simulink model "Q8"  (R2017a)
settings: Solver=ode4  StartTime=0.0  StopTime=10000  FixedStep=0.01  RelTol=1e-3  EnableMultiTasking=on
undefined symbols (not defined in the file): Cg, Cs, k, kc, kg, kr, sCon, Ta, u0
settings Model: Creator=Mikkel  LastModifiedBy=pebark
settings DataIOCC: LimitDataPoints=on  SaveFormat=Array  SignalLoggingSaveFormat=ModelDataLogs
settings OptimizationCC: ExpressionDepthLimit=2147483647  LifeSpan=inf
settings DebuggingCC: UnderspecifiedInitializationDetection=Classic  MergeDetectMultiDrivingBlocksExec=none  SolverPrmCheckMsg=warning  FcnCallInpInsideContextMsg=warning  StateNameClashWarn=warning  SFUnexpectedBacktrackingDiag=warning  SFNoUnconditionalDefaultTransitionDiag=warning  SFExecutionAtInitializationDiag=none
settings HardwareCC: ProdBitPerPointer=32  ProdBitPerSizeT=32  ProdBitPerPtrDiffT=32  ProdLargestAtomicFloat=None  ProdIntDivRoundTo=Undefined  ProdEndianess=Unspecified  ProdWordSize=32  ProdHWDeviceType=32-bit Generic
settings ModelReferenceCC: PropagateSignalLabelsOutOfModel=off
settings GRTTargetCC: TargetLangStandard=C89/C90 (ANSI)  GeneratePreprocessorConditionals=Disable all  CombineOutputUpdateFcns=off  GRTInterface=on
settings ConfigComp: CovMetricSettings=dw  CovHtmlReporting=on  CovSaveCumulativeToWorkspaceVar=on  CovSaveSingleToWorkspaceVar=on  CovExternalEMLEnable=off  CovSFcnEnable=off

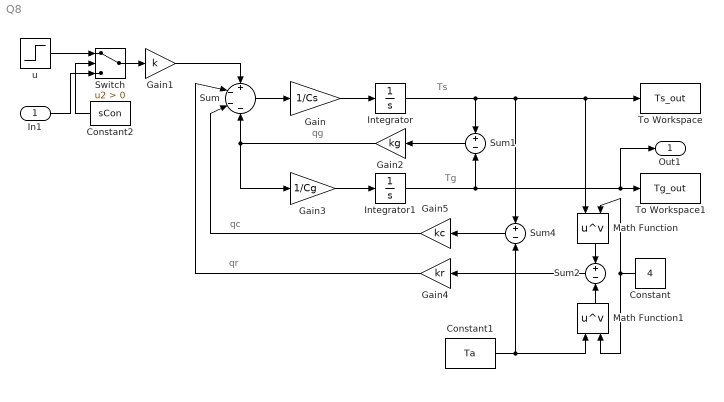
== system Q8 ==
  note: qg
  note: Ts
  note: Tg
  note: qr
  note: qc
  In1 : Inport
  Constant : Constant  Value=4
  Constant1 : Constant  Value=Ta
  Constant2 : Constant  Value=sCon
  Gain : Gain  Gain=1/Cs
  Gain1 : Gain  Gain=k
  Gain2 : Gain  Gain=kg
  Gain3 : Gain  Gain=1/Cg
  Gain4 : Gain  Gain=kr
  Gain5 : Gain  Gain=kc
  Integrator : Integrator  Priority=1  InitialCondition=473.15
  Integrator1 : Integrator  Priority=2  InitialCondition=298.15
  Math Function : Math  Operator=pow  SaturateOnIntegerOverflow=on
  Math Function1 : Math  Operator=pow  SaturateOnIntegerOverflow=on
  Sum : Sum  Inputs=+---
  Sum1 : Sum  Inputs=+-
  Sum2 : Sum  Inputs=+-
  Sum4 : Sum  Inputs=+-
  Switch : Switch  Criteria=u2 > Threshold
  To Workspace : ToWorkspace  VariableName=Ts_out  SaveFormat=Structure With Time  SampleTime=-1
  To Workspace1 : ToWorkspace  VariableName=Tg_out  SaveFormat=Structure With Time  SampleTime=-1
  u : Step  Time=0  Before=u0  After=u0  SampleTime=0
  Out1 : Outport
  wires:
  Gain/1 -> Integrator/1
  Sum/1 -> Gain/1
  Integrator/1 -> Sum1/1, Sum4/1, Math Function/1, To Workspace/1
  Sum1/1 -> Gain2/1
  Gain2/1 -> Gain3/1, Sum/4
  Gain3/1 -> Integrator1/1
  Integrator1/1 -> Sum1/2, To Workspace1/1, Out1/1
  Gain4/1 -> Sum/2
  Sum2/1 -> Gain4/1
  Gain1/1 -> Sum/1
  Math Function/1 -> Sum2/1
  Constant/1 -> Math Function/2, Math Function1/2
  Math Function1/1 -> Sum2/2
  Sum4/1 -> Gain5/1
  Gain5/1 -> Sum/3
  Switch/1 -> Gain1/1
  u/1 -> Switch/1
  In1/1 -> Switch/3
  Constant1/1 -> Sum4/2, Math Function1/1
  Constant2/1 -> Switch/2
